simulink model "lyskawaLab6_si"  (R2023b)
settings: Solver=VariableStepAuto  StartTime=0.0  StopTime=stopTime  MaxStep=0.01  RelTol=1e-3
values from neighbouring files (symbols this model uses):
  A1 = 1    [lyskawaLab6.m]
  a1 = Aw1 * sqrt(2*g/H1)    [lyskawaLab6.m]
  A2 = 1    [lyskawaLab6.m]
  a2 = Aw2 * sqrt(2*g/H2)    [lyskawaLab6.m]
  dfwe1 = 0    [lyskawaLab6.m]
  dfwe2 = 0.2 * fwe2max    [lyskawaLab6.m]
  fwe1_0 = 0.1*fwe1max    [lyskawaLab6.m]
  fwe2_0 = arrayfwe2_0(i)    [lyskawaLab6.m]
  h1_0 = fwe1_0/a1    [lyskawaLab6.m]
  h2_0 = arrayfwe2_0(i)/a2    [lyskawaLab6.m]
  t0 = 4    [lyskawaLab6.m]
settings Model: Creator=aleklyskawa  LastModifiedBy=aleklyskawa

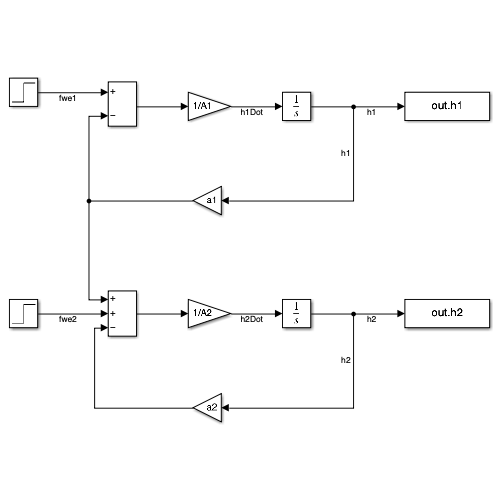
[thumbnail: Simulink's stored preview of the top-level diagram]
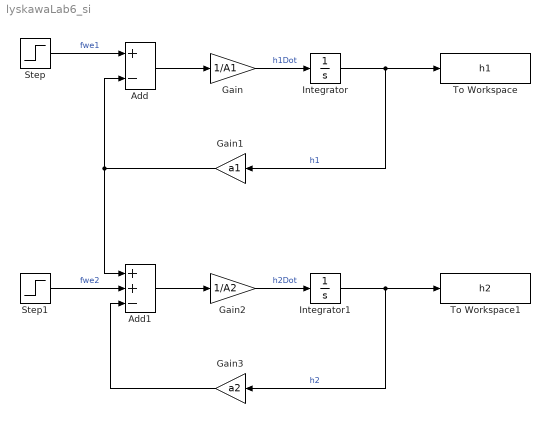
== system lyskawaLab6_si ==
  Add : Sum  Inputs=+-
  Add1 : Sum  Inputs=++-
  Gain : Gain  Gain=1/A1
  Gain1 : Gain  Gain=a1
  Gain2 : Gain  Gain=1/A2
  Gain3 : Gain  Gain=a2
  Integrator : Integrator  InitialCondition=h1_0
  Integrator1 : Integrator  InitialCondition=h2_0
  Step : Step  Time=t0  Before=fwe1_0  After=fwe1_0 + dfwe1  SampleTime=0
  Step1 : Step  Time=t0  Before=fwe2_0  After=fwe2_0 + dfwe2  SampleTime=0
  To Workspace : ToWorkspace  VariableName=h1  SampleTime=-1
  To Workspace1 : ToWorkspace  VariableName=h2  SampleTime=-1
  wires:
  Add/1 -> Gain/1
  Gain/1 -> Integrator/1  "h1Dot"
  Integrator/1 -> To Workspace/1, Gain1/1  "h1"
  Gain1/1 -> Add1/1, Add/2
  Step/1 -> Add/1  "fwe1"
  Integrator1/1 -> To Workspace1/1, Gain3/1  "h2"
  Add1/1 -> Gain2/1
  Gain3/1 -> Add1/3
  Gain2/1 -> Integrator1/1  "h2Dot"
  Step1/1 -> Add1/2  "fwe2"
